simulink model "Copy_of_accumulator_thermal_model"  (R2022a)
settings: Solver=VariableStepAuto  StartTime=0.0  StopTime=1900  RelTol=1e-7  AbsTol=1e-7
values from neighbouring files (symbols this model uses):
  cellInternalResis = .0018    (= 0.0018)    [Copy_of_Simulink_Setup.m]    (also in Simulink_Setup.m)
  startTempC = 23.5    [Copy_of_Simulink_Setup.m]    (also in HT06_Simulink_Setup.m = 23.3; Simulink_Setup.m)
  tabResis = 0.00009    (= 9e-05)    [Copy_of_Simulink_Setup.m]    (also in HT06_Simulink_Setup.m = 0.0001; Simulink_Setup.m)
libraries: fl_lib x26, nesl_utility x5, ee_lib x2
settings Model: Creator=elrii  LastModifiedBy=Pranav Nathan
settings SolverCC: AutoScaleAbsTol=off  AlgebraicLoopSolver=TrustRegion
settings DataIOCC: ReturnWorkspaceOutputsName=tp141c3138_a421_409b_bff7_0e00beb78378
settings DebuggingCC: UnconnectedInputMsg=warning  UnconnectedOutputMsg=warning  UnconnectedLineMsg=warning  SymbolicDimsDataTypeCodeGenerationDiagnostic=none  SFMachineParentedDataDiag=warning
settings SFSimCC: CustomCodeUndefinedFunction=UseInterfaceOnly
settings RTWCC: DLArmComputeVersion=19.05
settings SimscapeCC: SimscapeLogType=all  SimscapeLogSimulationStatistics=on  SimscapeLogDataHistory=10000

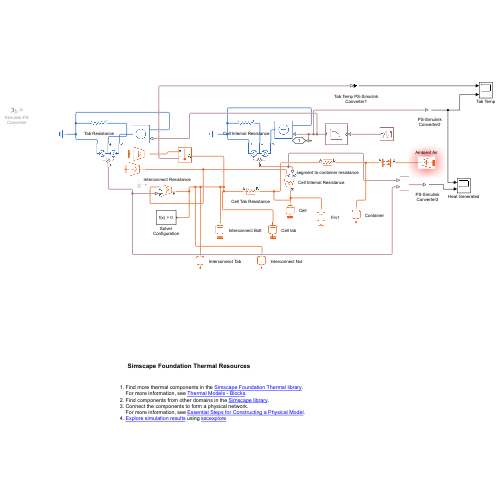
[thumbnail: Simulink's stored preview of the top-level diagram]
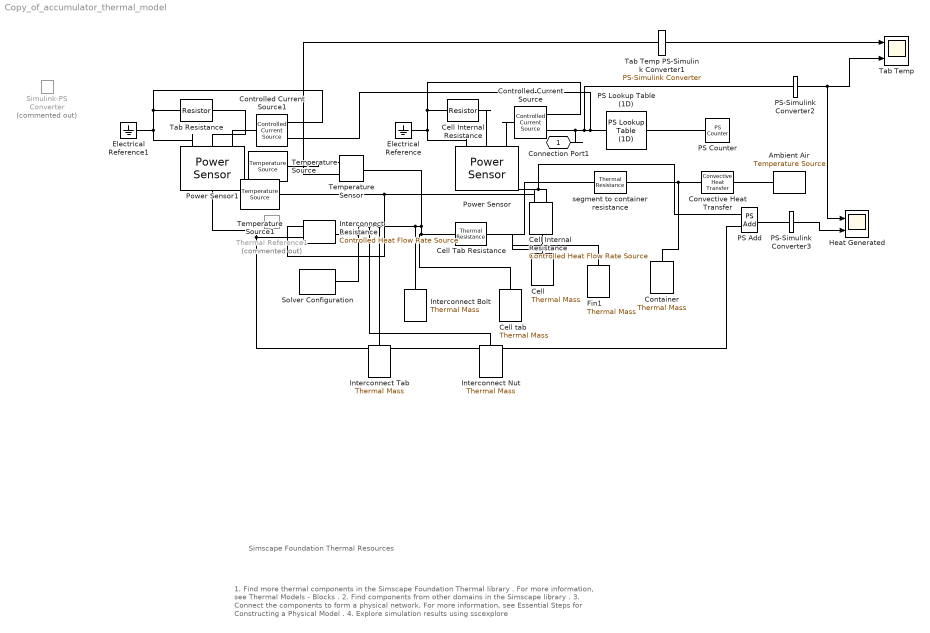
== system Copy_of_accumulator_thermal_model ==
  note: 1. Find more thermal components in the Simscape Foundation Thermal library .
      | For more information, see Thermal Models - Blocks .
      | 2. Find components from other domains in the Simscape library .
      | 3. Connect the components to form a physical network.
      | For more information, see Essential Steps for Constructing a Physical Model .
      | 4. Explore simulation results using sscexplore
  note: Simscape Foundation Thermal Resources
  " Fin1" : fl_lib/Thermal/Thermal Elements/Thermal Mass  mass=mFin kg  sp_heat=cAl J/kg/K  T_specify=on  T_priority=High  T=startTempC degC  T_nominal_specify=off  T_nominal_unit=K  T_nominal_value=1  Q_specify=off  Q_priority=None  Q=0 W  Q_nominal_specify=off  Q_nominal_unit=W  Q_nominal_value=1
      settings: SourceProductBaseCode=PW,SS,VE
  Ambient Air : fl_lib/Thermal/Thermal Sources/Temperature Source  temperature=ambientTempF degF
      settings: SourceProductBaseCode=PW,SS,VE
  "Cell " : fl_lib/Thermal/Thermal Elements/Thermal Mass  mass=mCell kg  sp_heat=cCell J/kg/K  T_specify=on  T_priority=High  T=startTempC degC  T_nominal_specify=off  T_nominal_unit=K  T_nominal_value=1  Q_specify=off  Q_priority=None  Q=0 W  Q_nominal_specify=off  Q_nominal_unit=W  Q_nominal_value=1
      settings: SourceProductBaseCode=PW,SS,VE
  Cell Internal Resistance : fl_lib/Thermal/Thermal Sources/Controlled Heat Flow Rate Source
      settings: SourceProductBaseCode=PW,SS,VE
  "Cell Internal Resistance " : fl_lib/Electrical/Electrical Elements/Resistor  R=cellInternalResis Ohm  i_specify=off  i_priority=None  i=0 A  i_nominal_specify=off  i_nominal_unit=A  i_nominal_value=1  v_specify=off  v_priority=None  v=0 V  v_nominal_specify=off  v_nominal_unit=V  v_nominal_value=1  mask(Resistor){}
      settings: SourceProductBaseCode=PW,SS,VE
  Cell Tab Resistance : fl_lib/Thermal/Thermal Elements/Thermal Resistance  resistance=R_tc K/W  T_specify=off  T_priority=None  T=0 K  T_nominal_specify=off  T_nominal_unit=K  T_nominal_value=1  Q_specify=off  Q_priority=None  Q=0 W  Q_nominal_specify=off  Q_nominal_unit=W  Q_nominal_value=1
      settings: SourceProductBaseCode=PW,SS,VE
  Cell tab : fl_lib/Thermal/Thermal Elements/Thermal Mass  mass=cellTabThermalMass kg  sp_heat=cCu J/kg/K  T_specify=on  T_priority=High  T=startTempC degC  T_nominal_specify=off  T_nominal_unit=K  T_nominal_value=1  Q_specify=off  Q_priority=None  Q=0 W  Q_nominal_specify=off  Q_nominal_unit=W  Q_nominal_value=1
      settings: SourceProductBaseCode=PW,SS,VE
  Container : fl_lib/Thermal/Thermal Elements/Thermal Mass  mass=0.05 kg  sp_heat=880 J/kg/K  T_specify=off  T_priority=High  T=300 K  T_nominal_specify=off  T_nominal_unit=K  T_nominal_value=1  Q_specify=off  Q_priority=None  Q=0 W  Q_nominal_specify=off  Q_nominal_unit=W  Q_nominal_value=1
      settings: SourceProductBaseCode=PW,SS,VE
  Controlled Current Source : fl_lib/Electrical/Electrical Sources/Controlled Current Source
      settings: SourceProductBaseCode=PW,SS,VE
  Controlled Current Source1 : fl_lib/Electrical/Electrical Sources/Controlled Current Source
      settings: SourceProductBaseCode=PW,SS,VE
  Convective Heat Transfer : fl_lib/Thermal/Thermal Elements/Convective Heat Transfer  area=convectionArea mm^2  heat_tr_coeff=10 W/(m^2 * K)  T_specify=off  T_priority=None  T=0 K  T_nominal_specify=off  T_nominal_unit=K  T_nominal_value=1  Q_specify=off  Q_priority=None  Q=0 W  Q_nominal_specify=off  Q_nominal_unit=W  Q_nominal_value=1
      settings: SourceProductBaseCode=PW,SS,VE
  Electrical Reference : fl_lib/Electrical/Electrical Elements/Electrical Reference
      settings: SourceProductBaseCode=PW,SS,VE
  Electrical Reference1 : fl_lib/Electrical/Electrical Elements/Electrical Reference
      settings: SourceProductBaseCode=PW,SS,VE
  Heat Generated : Scope  NumInputPorts=2
  Interconnect Bolt : fl_lib/Thermal/Thermal Elements/Thermal Mass  mass=mInterconnectBoltTotal kg  sp_heat=cSt J/kg/K  T_specify=on  T_priority=High  T=startTempC degC  T_nominal_specify=off  T_nominal_unit=K  T_nominal_value=1  Q_specify=off  Q_priority=None  Q=0 W  Q_nominal_specify=off  Q_nominal_unit=W  Q_nominal_value=1
      settings: SourceProductBaseCode=PW,SS,VE
  Interconnect Nut : fl_lib/Thermal/Thermal Elements/Thermal Mass  mass=mInterconnectNutTotal kg  sp_heat=cSt J/kg/K  T_specify=on  T_priority=High  T=startTempC degC  T_nominal_specify=off  T_nominal_unit=K  T_nominal_value=1  Q_specify=off  Q_priority=None  Q=0 W  Q_nominal_specify=off  Q_nominal_unit=W  Q_nominal_value=1
      settings: SourceProductBaseCode=PW,SS,VE
  Interconnect Resistance : fl_lib/Thermal/Thermal Sources/Controlled Heat Flow Rate Source
      settings: SourceProductBaseCode=PW,SS,VE
  Interconnect Tab : fl_lib/Thermal/Thermal Elements/Thermal Mass  mass=mInterconnect kg  sp_heat=cAl J/kg/K  T_specify=on  T_priority=High  T=startTempC degC  T_nominal_specify=off  T_nominal_unit=K  T_nominal_value=1  Q_specify=off  Q_priority=None  Q=0 W  Q_nominal_specify=off  Q_nominal_unit=W  Q_nominal_value=1
      settings: SourceProductBaseCode=PW,SS,VE
  PS Add : fl_lib/Physical Signals/Functions/PS Add
      settings: SourceProductBaseCode=PW,SS,VE
  PS Counter : fl_lib/Physical Signals/Sources/PS Counter  sample_time=1 s  init_val=1  reset_val=0  max_val=100000
      settings: SourceProductBaseCode=PW,SS,VE  InternalSimscapePortConfiguration="{\"Bottom\":[],\"Left\":[],\"Right\":[{\"id\":\"Y\",\"label\":\"Y\",\"type\":\"output\"}],\"Top\":[]}"
  PS Lookup Table (1D) : fl_lib/Physical Signals/Lookup Tables/PS Lookup Table (1D)  x=time  f=current  interp_method=simscape.enum.interpolation.linear  extrap_method=simscape.enum.extrapolation.linear
      settings: SourceProductBaseCode=PW,SS,VE
  PS-Simulink Converter2 : nesl_utility/PS-Simulink Converter  PhysicalDomain=network_engine_domain  SubClassName=ps_output  LeftPortType=input  RightPortType=output  PseudoPeriodic=off  Frequencies=[]  VectorFormat=1-D array  Unit=inherit  AffineConversion=off
      settings: SourceProductBaseCode=SS,PW,VE
  PS-Simulink Converter3 : nesl_utility/PS-Simulink Converter  PhysicalDomain=network_engine_domain  SubClassName=ps_output  LeftPortType=input  RightPortType=output  PseudoPeriodic=off  Frequencies=[]  VectorFormat=1-D array  Unit=inherit  AffineConversion=off
      settings: SourceProductBaseCode=SS,PW,VE
  Power Sensor : ee_lib/Sensors & Transducers/Power Sensor  measurement_type=1  averaging_period=1e-4 s
      settings: SourceProductBaseCode=PS
  Power Sensor1 : ee_lib/Sensors & Transducers/Power Sensor  measurement_type=1  averaging_period=1e-4 s
      settings: SourceProductBaseCode=PS
  Simulink-PS Converter : nesl_utility/Simulink-PS Converter  Commented=on  PhysicalDomain=network_engine_domain  SubClassName=ps_input  LeftPortType=input  RightPortType=output  PseudoPeriodic=off  Frequencies=[]  NoiseDistribution=none  NoiseParameters=[]  Unit=1  AffineConversion=off  FilteringAndDerivatives=provide  SimscapeFilterOrder=1  InputFilterTimeConstant=0.001  UdotUserProvided=0
      settings: SourceProductBaseCode=SS,PW,VE
  Solver Configuration : nesl_utility/Solver Configuration  PhysicalDomain=network_engine_domain  SubClassName=solver  LeftPortType=input  RightPortType=generic  Tones=[]  Harmonics=[]  SimulateNoise=off  Profile=off  UseLocalSampling=off  EnableSwitchedLinearOptims=on  FrequencyDomain=off  UseCCode=off  RelTol=0.001  AbsTol=1e-06  MinStep=1e-09  ToWorkspace=off  RevertToSquareIcSolve=off  NumHomotopyIterations=100  PhasorMode=off  PhasorModeNumHarmonics=1  IndexReductionMethod=DerivativeReplacement  DoDC=off  ResidualTolerance=1e-011  UseLocalSolver=off  LocalSolverChoice=NE_BACKWARD_EULER_ADVANCER  LocalSolverSampleTime=0.001  DoFixedCost=off  MaxNonlinIter=3  MaxModeIter=2  ComputeImpulses=off  ImpulseIterations=2  LinearAlgebra=auto  LinearAlgebraNumThread=0  EquationFormulation=NE_TIME_EF  DelaysMemoryBudget=1024  AutomaticFiltering=on  FilteringTimeConstant=0.001  PartitionStorageMethod=AS_NEEDED  PartitionMemoryBudget=1024  PartitionMethod=ROBUST
      settings: SourceProductBaseCode=SS,PW,VE
  Tab Resistance : fl_lib/Electrical/Electrical Elements/Resistor  R=tabResis Ohm  i_specify=off  i_priority=None  i=0 A  i_nominal_specify=off  i_nominal_unit=A  i_nominal_value=1  v_specify=off  v_priority=None  v=0 V  v_nominal_specify=off  v_nominal_unit=V  v_nominal_value=1  mask(Resistor){}
      settings: SourceProductBaseCode=PW,SS,VE
  Tab Temp : Scope  NumInputPorts=2
  Tab Temp PS-Simulink Converter1 : nesl_utility/PS-Simulink Converter  PhysicalDomain=network_engine_domain  SubClassName=ps_output  LeftPortType=input  RightPortType=output  PseudoPeriodic=off  Frequencies=[]  VectorFormat=1-D array  Unit=inherit  AffineConversion=off
      settings: SourceProductBaseCode=SS,PW,VE
  Temperature Sensor : fl_lib/Thermal/Thermal Sensors/Temperature Sensor
      settings: SourceProductBaseCode=PW,SS,VE
  Temperature Source : fl_lib/Thermal/Thermal Sources/Temperature Source  temperature=0 degC
      settings: SourceProductBaseCode=PW,SS,VE
  Temperature Source1 : fl_lib/Thermal/Thermal Sources/Temperature Source  temperature=0 degC
      settings: SourceProductBaseCode=PW,SS,VE
  Thermal Reference1 : fl_lib/Thermal/Thermal Elements/Thermal Reference  Commented=on
      settings: SourceProductBaseCode=PW,SS,VE
  segment to container resistance : fl_lib/Thermal/Thermal Elements/Thermal Resistance  resistance=R_cb K/W  T_specify=off  T_priority=None  T=0 K  T_nominal_specify=off  T_nominal_unit=K  T_nominal_value=1  Q_specify=off  Q_priority=None  Q=0 W  Q_nominal_specify=off  Q_nominal_unit=W  Q_nominal_value=1
      settings: SourceProductBaseCode=PW,SS,VE
  Connection Port1 : PMIOPort  Side=Left
  wires:
  PS-Simulink Converter2/1 -> Heat Generated/1, Tab Temp/2
  PS-Simulink Converter3/1 -> Heat Generated/2
  Tab Temp PS-Simulink Converter1/1 -> Tab Temp/1
  connections:
  Cell Internal Resistance/LConn1 -- segment to container resistance/LConn1 -- Cell Tab Resistance/RConn1 -- "Cell "/LConn1 -- " Fin1"/LConn1
  Interconnect Resistance/LConn1 -- Interconnect Bolt/LConn1 -- Temperature Sensor/LConn1 -- Cell Tab Resistance/LConn1 -- Cell tab/LConn1 -- Interconnect Tab/LConn1 -- Interconnect Nut/LConn1 -- Solver Configuration/RConn1
  Controlled Current Source/LConn1 -- Power Sensor/LConn1
  "Cell Internal Resistance "/LConn1 -- Power Sensor/LConn2
  Power Sensor/LConn3 -- Electrical Reference/LConn1 -- Controlled Current Source/RConn2 -- "Cell Internal Resistance "/RConn1
  Controlled Current Source1/RConn2 -- Power Sensor1/LConn3 -- Electrical Reference1/LConn1 -- Tab Resistance/RConn1
  Tab Resistance/LConn1 -- Power Sensor1/LConn2
  Controlled Current Source1/LConn1 -- Power Sensor1/LConn1
  Power Sensor1/RConn1 -- PS Add/LConn2 -- Interconnect Resistance/RConn1
  Cell Internal Resistance/RConn2 -- Temperature Source1/LConn1 -- Interconnect Resistance/RConn2
  segment to container resistance/RConn1 -- Container/LConn1 -- Convective Heat Transfer/LConn1
  Ambient Air/LConn1 -- Convective Heat Transfer/RConn1
  Controlled Current Source/RConn1 -- Connection Port1/RConn1 -- PS-Simulink Converter2/LConn1 -- PS Lookup Table (1D)/RConn1 -- Controlled Current Source1/RConn1
  PS Counter/RConn1 -- PS Lookup Table (1D)/LConn1
  Temperature Source/LConn1 -- Temperature Sensor/RConn1
  Cell Internal Resistance/RConn1 -- PS Add/LConn1 -- Power Sensor/RConn1
  PS Add/RConn1 -- PS-Simulink Converter3/LConn1
  Tab Temp PS-Simulink Converter1/LConn1 -- Temperature Sensor/RConn2
